simulink model "lorenz3d"  (R2026b)
settings Model: ExtModeTrigMode=oneshot  ExtModeArmWhenConnect=off  Creator=The MathWorks Inc.  LastModifiedBy=gcampa

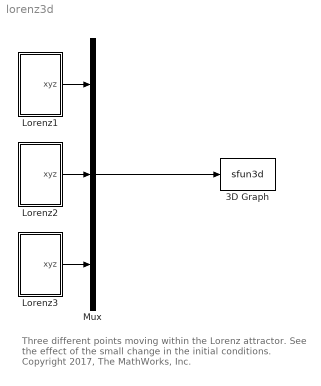
== system lorenz3d ==
  note: Three different points moving within the Lorenz attractor.
      | See the effect of the small change in the initial conditions.
      | Copyright 2017, The MathWorks, Inc.
  3D Graph : M-S-Function  LoadFcn=if exist('sfun3d','file'), sfun3d([],'LoadBlock'); end  FunctionName=sfun3d  Parameters=ax,T,np,cp,gd,ls,mk,mx,hd,tb  mask(3D Graph){np=3, ax=[-30 30 -30 30 0 50], mx=2000, T=0.01, cp=[370 -234 -207], gd=on, hd=on, tb=off, ls=-, mk=none}
      mask prompts: np "Number of moving points (lines)"; ax "Range: [xmin xmax  ymin ymax zmin zmax]"; mx "Max number of points in each line"; T "Sampling Time"; cp "Camera position (use [0 0 1] for 2D XY view)"; gd "Grid (on|off)"; hd "HeadMarkers (on|off)"; tb "Toolbar (on|off)"; ls "LineStyle"; mk "LineMarker"
      mask help:
      | This block plots the position of several points in the XYZ space. The input contains the coordinates of all the points (x1,y1,z1,x2,y2,z2,...).
      | The number of moving points (lines), the XYZ ranges, sampling time, camera position, and grid (among other things) can be set as mask parameters.
      settings: CopyFcn=if exist('sfun3d','file'), sfun3d([],'CopyBlock'); end  DeleteFcn=if exist('sfun3d','file'), sfun3d([],'DeleteBlock'); end  NameChangeFcn=if exist('sfun3d','file'), sfun3d([],'NameChange'); end
      mask Help:
      | This block plots the position of several points in the XYZ space. The input contains the coordinates of all the points (x1,y1,z1,x2,y2,z2,...).
      | The number of moving points (lines), the XYZ ranges, sampling time, camera position, and grid (among other things) can be set as mask parameters.
      mask TypeOptions ls: - | -- | : | -. | none
      mask TypeOptions mk: none | . | + | o | * | x | square | diamond | v | ^ | > | < | pentagram | hexagram
      mask Display: t=linspace(0,2*pi,50); plot(sin(2*t),sin(3*t+pi/2));
  Lorenz1 : Subsystem  mask(Lorenz Attractor System){s=10, r=28, b=2+2/3, xyz0=[1 1 1]}
      mask prompts: s "sigma"; r "rho"; b "beta"; xyz0 "Initial State (x0, y0, y0)"
      mask help:
      | This autonomous system generates the lorentz attractor:
      | xdot=sigma*(x-y); ydot=rho*x-y-x*z; zdot=-beta*z+x*y;
      | Parameters and initial state can be selected from the mask.
      mask Help:
      | This autonomous system generates the lorentz attractor.
      | Parameters and initial state can be selected from the mask.
      | <p>
      | The system equations are:
      | xdot = sigma*(x-y),
      | ydot = rho*x-y-x*z,
      | zdot = -beta*z+x*y,
  Lorenz2 : Subsystem  mask(Lorenz Attractor System){s=10, r=28, b=2+2/3, xyz0=[2 2 2]}
      mask prompts: s "sigma"; r "rho"; b "beta"; xyz0 "Initial State (x0, y0, y0)"
      mask help:
      | This autonomous system generates the lorentz attractor:
      | xdot=sigma*(x-y); ydot=rho*x-y-x*z; zdot=-beta*z+x*y;
      | Parameters and initial state can be selected from the mask.
      mask Help:
      | This autonomous system generates the lorentz attractor.
      | Parameters and initial state can be selected from the mask.
      | <p>
      | The system equations are:
      | xdot = sigma*(x-y),
      | ydot = rho*x-y-x*z,
      | zdot = -beta*z+x*y,
  Lorenz3 : Subsystem  mask(Lorenz Attractor System){s=10, r=28, b=2+2/3, xyz0=[3 3 3]}
      mask prompts: s "sigma"; r "rho"; b "beta"; xyz0 "Initial State (x0, y0, y0)"
      mask help:
      | This autonomous system generates the lorentz attractor:
      | xdot=sigma*(x-y); ydot=rho*x-y-x*z; zdot=-beta*z+x*y;
      | Parameters and initial state can be selected from the mask.
      mask Help:
      | This autonomous system generates the lorentz attractor.
      | Parameters and initial state can be selected from the mask.
      | <p>
      | The system equations are:
      | xdot = sigma*(x-y),
      | ydot = rho*x-y-x*z,
      | zdot = -beta*z+x*y,
  Mux : Mux  Inputs=[3 3 3]
  wires:
  Lorenz1/1(xyz) -> Mux/1
  Lorenz2/1(xyz) -> Mux/2
  Lorenz3/1(xyz) -> Mux/3
  Mux/1 -> 3D Graph/1

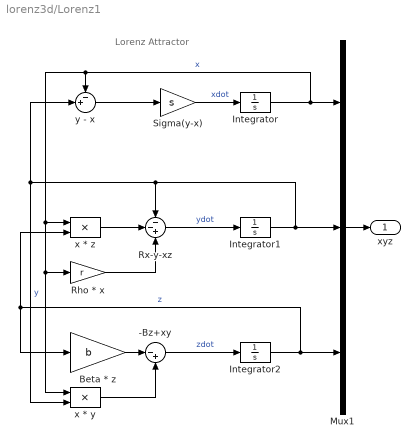
== system lorenz3d/Lorenz1 ==
  note: Lorenz Attractor
  -Bz+xy : Sum  Inputs=|-+  InputSameDT=on  SaturateOnIntegerOverflow=on  OutDataTypeStr=Inherit: Same as first input
  Beta * z : Gain  Gain=b  SaturateOnIntegerOverflow=on  OutDataTypeStr=Inherit: Same as input  ParamDataTypeStr=Inherit: Same as input
  Integrator : Integrator  InitialCondition=xyz0(1)
  Integrator1 : Integrator  InitialCondition=xyz0(2)
  Integrator2 : Integrator  InitialCondition=xyz0(3)
  Mux1 : Mux  Inputs=3
  Rho * x : Gain  Gain=r  SaturateOnIntegerOverflow=on  OutDataTypeStr=Inherit: Same as input  ParamDataTypeStr=Inherit: Same as input
  Rx-y-xz : Sum  Inputs=--+  InputSameDT=on  SaturateOnIntegerOverflow=on  OutDataTypeStr=Inherit: Same as first input
  Sigma(y-x) : Gain  Gain=s  SaturateOnIntegerOverflow=on  OutDataTypeStr=Inherit: Same as input  ParamDataTypeStr=Inherit: Same as input
  x * y : Product  InputSameDT=on  RndMeth=Zero  SaturateOnIntegerOverflow=on  OutDataTypeStr=Inherit: Same as first input
  x * z : Product  InputSameDT=on  RndMeth=Zero  SaturateOnIntegerOverflow=on  OutDataTypeStr=Inherit: Same as first input
  y - x : Sum  Inputs=-+|  InputSameDT=on  SaturateOnIntegerOverflow=on  OutDataTypeStr=Inherit: Same as first input
  xyz : Outport
  wires:
  Sigma(y-x)/1 -> Integrator/1  "xdot"
  y - x/1 -> Sigma(y-x)/1
  Rx-y-xz/1 -> Integrator1/1  "ydot"
  x * z/1 -> Rx-y-xz/2
  Integrator2/1 -> x * z/2, Beta * z/1, Mux1/3  "z"
  Integrator1/1 -> Rx-y-xz/1, y - x/2, x * y/2, Mux1/2  "y"
  Integrator/1 -> y - x/1, x * z/1, Rho * x/1, x * y/1, Mux1/1  "x"
  -Bz+xy/1 -> Integrator2/1  "zdot"
  Beta * z/1 -> -Bz+xy/1
  x * y/1 -> -Bz+xy/2
  Mux1/1 -> xyz/1
  Rho * x/1 -> Rx-y-xz/3

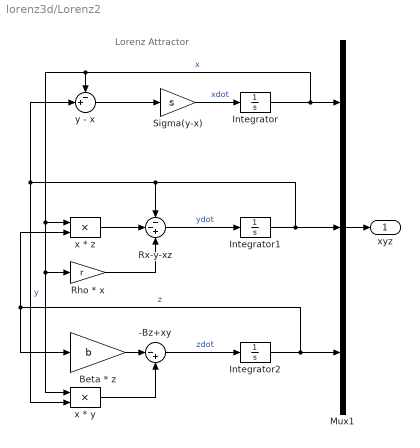
== system lorenz3d/Lorenz2 ==
  note: Lorenz Attractor
  -Bz+xy : Sum  Inputs=|-+  InputSameDT=on  SaturateOnIntegerOverflow=on  OutDataTypeStr=Inherit: Same as first input
  Beta * z : Gain  Gain=b  SaturateOnIntegerOverflow=on  OutDataTypeStr=Inherit: Same as input  ParamDataTypeStr=Inherit: Same as input
  Integrator : Integrator  InitialCondition=xyz0(1)
  Integrator1 : Integrator  InitialCondition=xyz0(2)
  Integrator2 : Integrator  InitialCondition=xyz0(3)
  Mux1 : Mux  Inputs=3
  Rho * x : Gain  Gain=r  SaturateOnIntegerOverflow=on  OutDataTypeStr=Inherit: Same as input  ParamDataTypeStr=Inherit: Same as input
  Rx-y-xz : Sum  Inputs=--+  InputSameDT=on  SaturateOnIntegerOverflow=on  OutDataTypeStr=Inherit: Same as first input
  Sigma(y-x) : Gain  Gain=s  SaturateOnIntegerOverflow=on  OutDataTypeStr=Inherit: Same as input  ParamDataTypeStr=Inherit: Same as input
  x * y : Product  InputSameDT=on  RndMeth=Zero  SaturateOnIntegerOverflow=on  OutDataTypeStr=Inherit: Same as first input
  x * z : Product  InputSameDT=on  RndMeth=Zero  SaturateOnIntegerOverflow=on  OutDataTypeStr=Inherit: Same as first input
  y - x : Sum  Inputs=-+|  InputSameDT=on  SaturateOnIntegerOverflow=on  OutDataTypeStr=Inherit: Same as first input
  xyz : Outport
  wires:
  Mux1/1 -> xyz/1
  x * y/1 -> -Bz+xy/2
  Beta * z/1 -> -Bz+xy/1
  -Bz+xy/1 -> Integrator2/1  "zdot"
  Integrator/1 -> Mux1/1, x * y/1, Rho * x/1, x * z/1, y - x/1  "x"
  Integrator1/1 -> Mux1/2, x * y/2, y - x/2, Rx-y-xz/1  "y"
  Integrator2/1 -> Mux1/3, Beta * z/1, x * z/2  "z"
  x * z/1 -> Rx-y-xz/2
  Rx-y-xz/1 -> Integrator1/1  "ydot"
  y - x/1 -> Sigma(y-x)/1
  Sigma(y-x)/1 -> Integrator/1  "xdot"
  Rho * x/1 -> Rx-y-xz/3

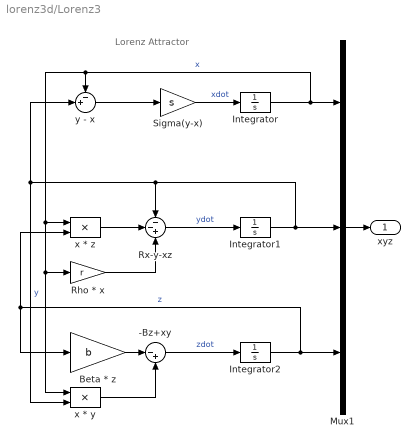
== system lorenz3d/Lorenz3 ==
  note: Lorenz Attractor
  -Bz+xy : Sum  Inputs=|-+  InputSameDT=on  SaturateOnIntegerOverflow=on  OutDataTypeStr=Inherit: Same as first input
  Beta * z : Gain  Gain=b  SaturateOnIntegerOverflow=on  OutDataTypeStr=Inherit: Same as input  ParamDataTypeStr=Inherit: Same as input
  Integrator : Integrator  InitialCondition=xyz0(1)
  Integrator1 : Integrator  InitialCondition=xyz0(2)
  Integrator2 : Integrator  InitialCondition=xyz0(3)
  Mux1 : Mux  Inputs=3
  Rho * x : Gain  Gain=r  SaturateOnIntegerOverflow=on  OutDataTypeStr=Inherit: Same as input  ParamDataTypeStr=Inherit: Same as input
  Rx-y-xz : Sum  Inputs=--+  InputSameDT=on  SaturateOnIntegerOverflow=on  OutDataTypeStr=Inherit: Same as first input
  Sigma(y-x) : Gain  Gain=s  SaturateOnIntegerOverflow=on  OutDataTypeStr=Inherit: Same as input  ParamDataTypeStr=Inherit: Same as input
  x * y : Product  InputSameDT=on  RndMeth=Zero  SaturateOnIntegerOverflow=on  OutDataTypeStr=Inherit: Same as first input
  x * z : Product  InputSameDT=on  RndMeth=Zero  SaturateOnIntegerOverflow=on  OutDataTypeStr=Inherit: Same as first input
  y - x : Sum  Inputs=-+|  InputSameDT=on  SaturateOnIntegerOverflow=on  OutDataTypeStr=Inherit: Same as first input
  xyz : Outport
  wires:
  Sigma(y-x)/1 -> Integrator/1  "xdot"
  y - x/1 -> Sigma(y-x)/1
  Rx-y-xz/1 -> Integrator1/1  "ydot"
  x * z/1 -> Rx-y-xz/2
  Integrator2/1 -> x * z/2, Beta * z/1, Mux1/3  "z"
  Integrator1/1 -> Rx-y-xz/1, y - x/2, x * y/2, Mux1/2  "y"
  Integrator/1 -> y - x/1, x * z/1, Rho * x/1, x * y/1, Mux1/1  "x"
  -Bz+xy/1 -> Integrator2/1  "zdot"
  Beta * z/1 -> -Bz+xy/1
  x * y/1 -> -Bz+xy/2
  Mux1/1 -> xyz/1
  Rho * x/1 -> Rx-y-xz/3
